simulink model "Chap5_DemodFixdt"  (R2015a)
settings: Solver=ode45  StartTime=0.0  StopTime=10  RelTol=1e-3
undefined symbols (not defined in the file or in its folder): clock
libraries: commsink2 x2, commchan3 x1, commrandsrc2 x1, commdigbbndam3 x1
settings Model: FPTRunName=FPA_Reference  Creator=Administrator  LastModifiedBy=Administrator
settings HardwareCC: ProdHWDeviceType=ASIC/FPGA->ASIC/FPGA  TargetLongLongMode=on  TargetIntDivRoundTo=Zero  TargetEndianess=LittleEndian  TargetHWDeviceType=MATLAB Host  ProdEqTarget=off

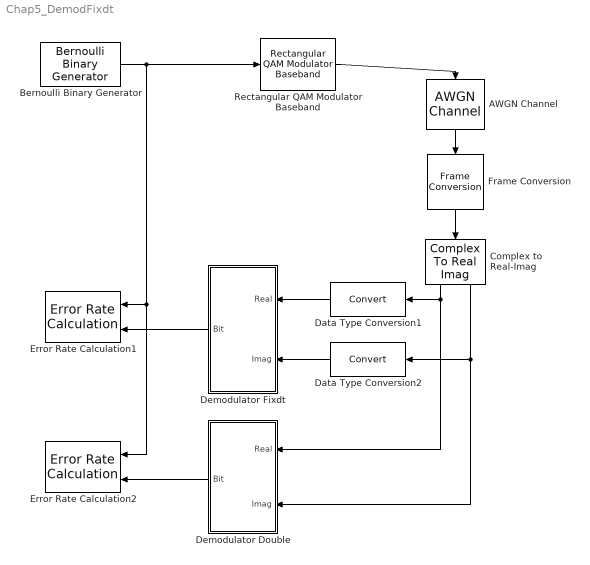
== system Chap5_DemodFixdt ==
  AWGN Channel : commchan3/AWGN Channel  InputProcessing=Columns as channels (frame based)  seed=round(200 * sum(clock))  noiseMode="Signal to noise ratio  (SNR)"  EbNodB=10  EsNodB=10  SNRdB=7  bitsPerSym=1  Ps=1  Tsym=1  variance=1
  Bernoulli Binary Generator : commrandsrc2/Bernoulli Binary Generator  P=0.5  seed=round(100 * sum(clock))  Ts=0.25e-6  frameBased=on  sampPerFrame=4  orient=off  outDataType=boolean
  Complex to Real-Imag : ComplexToRealImag
  Data Type Conversion1 : DataTypeConversion
  Data Type Conversion2 : DataTypeConversion
  Demodulator Double : Subsystem
  Demodulator Fixdt : Subsystem  MinMaxOverflowLogging=MinMaxAndOverflow
  Error Rate Calculation1 : commsink2/Error Rate Calculation  N=0  st_delay=0  cp_mode=Entire frame  subframe=[]  PMode=Workspace  WsName=ErrorVecFixdt  RsMode2=off  stop=off  numErr=100  maxBits=1e6
  Error Rate Calculation2 : commsink2/Error Rate Calculation  N=0  st_delay=0  cp_mode=Entire frame  subframe=[]  PMode=Workspace  WsName=ErrorVecDouble  RsMode2=off  stop=off  numErr=100  maxBits=1e6
  Frame Conversion : FrameConversion  OutFrame=Sample-based
  Rectangular QAM Modulator Baseband : commdigbbndam3/Rectangular QAM Modulator Baseband  M=16  InType=Bit  Enc=Gray  Mapping=[0:15]  PowType=Average Power  MinDist=2  AvgPow=1  PeakPow=1  Ph=0  outDtype=double  outWordLen=16  outUDDataType=sfix(16)  outFracLenMode=Best precision  outFracLen=15
  wires:
  Bernoulli Binary Generator/1 -> Error Rate Calculation2/1, Error Rate Calculation1/1, Rectangular QAM Modulator Baseband/1
  Rectangular QAM Modulator Baseband/1 -> AWGN Channel/1
  AWGN Channel/1 -> Frame Conversion/1
  Complex to Real-Imag/1 -> Demodulator Double/1(Real), Data Type Conversion1/1
  Complex to Real-Imag/2 -> Demodulator Double/2(Imag), Data Type Conversion2/1
  Frame Conversion/1 -> Complex to Real-Imag/1
  Demodulator Fixdt/1(Bit) -> Error Rate Calculation1/2
  Data Type Conversion1/1 -> Demodulator Fixdt/1(Real)
  Data Type Conversion2/1 -> Demodulator Fixdt/2(Imag)
  Demodulator Double/1(Bit) -> Error Rate Calculation2/2

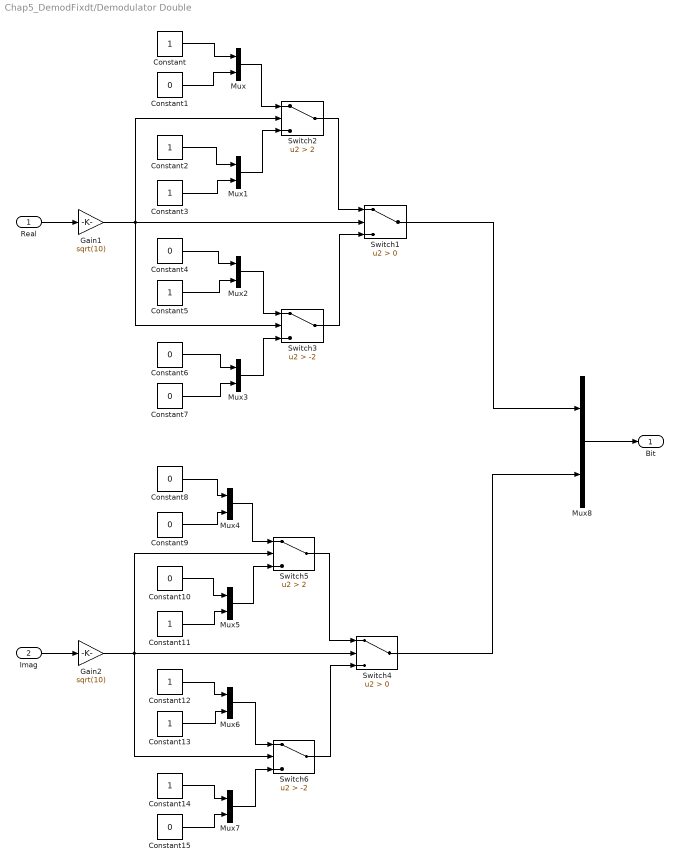
== system Chap5_DemodFixdt/Demodulator Double ==
  Real : Inport
  Imag : Inport  Port=2
  Constant{,2..3,5,11..14} (8 alike) : Constant  OutDataTypeStr=boolean
  Constant{1,4,6..10,15} (8 alike) : Constant  Value=0  OutDataTypeStr=boolean
  Gain1 : Gain  Gain=sqrt(10)
  Gain2 : Gain  Gain=sqrt(10)
  Mux{,1..8} (9 alike) : Mux  Inputs=2
  Switch1 : Switch  Criteria=u2 > Threshold
  Switch2 : Switch  Criteria=u2 > Threshold  Threshold=2
  Switch3 : Switch  Criteria=u2 > Threshold  Threshold=-2
  Switch4 : Switch  Criteria=u2 > Threshold
  Switch5 : Switch  Criteria=u2 > Threshold  Threshold=2
  Switch6 : Switch  Criteria=u2 > Threshold  Threshold=-2
  Bit : Outport
  wires:
  Constant/1 -> Mux/1
  Real/1 -> Gain1/1
  Constant2/1 -> Mux1/1
  Switch2/1 -> Switch1/1
  Constant7/1 -> Mux3/2
  Constant1/1 -> Mux/2
  Constant6/1 -> Mux3/1
  Mux/1 -> Switch2/1
  Constant3/1 -> Mux1/2
  Mux3/1 -> Switch3/3
  Switch3/1 -> Switch1/3
  Constant4/1 -> Mux2/1
  Mux2/1 -> Switch3/1
  Mux1/1 -> Switch2/3
  Constant5/1 -> Mux2/2
  Switch1/1 -> Mux8/1
  Constant14/1 -> Mux7/1
  Constant10/1 -> Mux5/1
  Imag/1 -> Gain2/1
  Mux5/1 -> Switch5/3
  Mux6/1 -> Switch6/1
  Constant9/1 -> Mux4/2
  Constant15/1 -> Mux7/2
  Switch4/1 -> Mux8/2
  Switch6/1 -> Switch4/3
  Mux7/1 -> Switch6/3
  Constant11/1 -> Mux5/2
  Mux4/1 -> Switch5/1
  Switch5/1 -> Switch4/1
  Constant8/1 -> Mux4/1
  Constant13/1 -> Mux6/2
  Constant12/1 -> Mux6/1
  Gain1/1 -> Switch3/2, Switch2/2, Switch1/2
  Gain2/1 -> Switch5/2, Switch6/2, Switch4/2
  Mux8/1 -> Bit/1

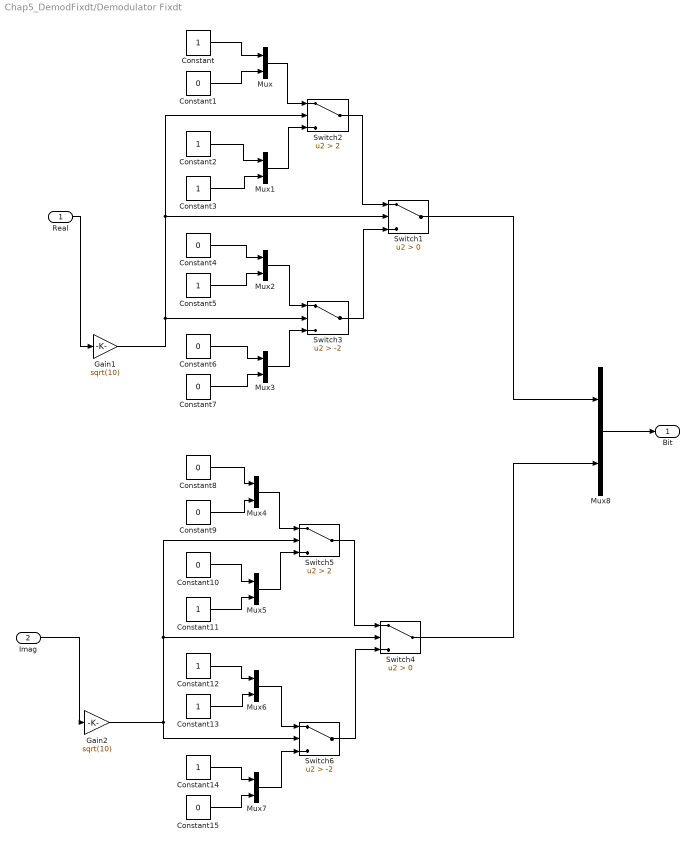
== system Chap5_DemodFixdt/Demodulator Fixdt ==
  Real : Inport  OutDataTypeStr=fixdt(1,16,13)  LockScale=on
  Imag : Inport  Port=2  OutDataTypeStr=fixdt(1,16,13)  LockScale=on
  Constant{,2..3,5,11..14} (8 alike) : Constant  OutDataTypeStr=boolean
  Constant{1,4,6..10,15} (8 alike) : Constant  Value=0  OutDataTypeStr=boolean
  Gain1 : Gain  Gain=sqrt(10)  OutDataTypeStr=fixdt(1,16,12)
  Gain2 : Gain  Gain=sqrt(10)  OutDataTypeStr=fixdt(1,16,12)
  Mux{,1..8} (9 alike) : Mux  Inputs=2
  Switch1 : Switch  Criteria=u2 > Threshold
  Switch2 : Switch  Criteria=u2 > Threshold  Threshold=2
  Switch3 : Switch  Criteria=u2 > Threshold  Threshold=-2
  Switch4 : Switch  Criteria=u2 > Threshold
  Switch5 : Switch  Criteria=u2 > Threshold  Threshold=2
  Switch6 : Switch  Criteria=u2 > Threshold  Threshold=-2
  Bit : Outport
  wires:
  Constant/1 -> Mux/1
  Real/1 -> Gain1/1
  Constant2/1 -> Mux1/1
  Switch2/1 -> Switch1/1
  Constant7/1 -> Mux3/2
  Constant1/1 -> Mux/2
  Constant6/1 -> Mux3/1
  Mux/1 -> Switch2/1
  Constant3/1 -> Mux1/2
  Mux3/1 -> Switch3/3
  Switch3/1 -> Switch1/3
  Constant4/1 -> Mux2/1
  Mux2/1 -> Switch3/1
  Mux1/1 -> Switch2/3
  Constant5/1 -> Mux2/2
  Switch1/1 -> Mux8/1
  Constant14/1 -> Mux7/1
  Constant10/1 -> Mux5/1
  Imag/1 -> Gain2/1
  Mux5/1 -> Switch5/3
  Mux6/1 -> Switch6/1
  Constant9/1 -> Mux4/2
  Constant15/1 -> Mux7/2
  Switch4/1 -> Mux8/2
  Switch6/1 -> Switch4/3
  Mux7/1 -> Switch6/3
  Constant11/1 -> Mux5/2
  Mux4/1 -> Switch5/1
  Switch5/1 -> Switch4/1
  Constant8/1 -> Mux4/1
  Constant13/1 -> Mux6/2
  Constant12/1 -> Mux6/1
  Gain1/1 -> Switch2/2, Switch1/2, Switch3/2
  Gain2/1 -> Switch5/2, Switch4/2, Switch6/2
  Mux8/1 -> Bit/1
